simulink model "VT_Bridge"  (Simulink 7.5)
settings: Solver=ode45  StartTime=0.0  StopTime=10.0  RelTol=1e-3
libraries: powerlib x4
settings Model: Creator=lm  LastModifiedBy=lm

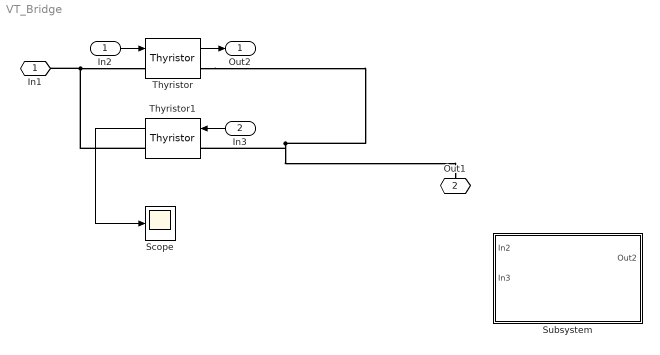
== system VT_Bridge ==
  In2 : Inport
  In3 : Inport  Port=2
  Scope : Scope
  Subsystem : Subsystem
  Thyristor : powerlib/Power Electronics/Thyristor  DialogController=POWERSYS.PowerSysDialog  SystemSampleTime=-1  Ron=0.001  Lon=0  Vf=0.8  IC=0  Rs=500  Cs=250e-9  Measurements=on
  Thyristor1 : powerlib/Power Electronics/Thyristor  DialogController=POWERSYS.PowerSysDialog  SystemSampleTime=-1  Ron=0.001  Lon=0  Vf=0.8  IC=0  Rs=500  Cs=250e-9  Measurements=on
  In1 : PMIOPort  Port=1  Side=Left
  Out1 : PMIOPort  Port=2  Side=Right
  Out2 : Outport
  wires:
  In3/1 -> Thyristor1/1
  Thyristor/1 -> Out2/1
  In2/1 -> Thyristor/1
  Thyristor1/1 -> Scope/1
  connections:
  Thyristor1/LConn1 -- Out1/RConn1 -- Thyristor/RConn1
  Thyristor1/RConn1 -- In1/RConn1 -- Thyristor/LConn1

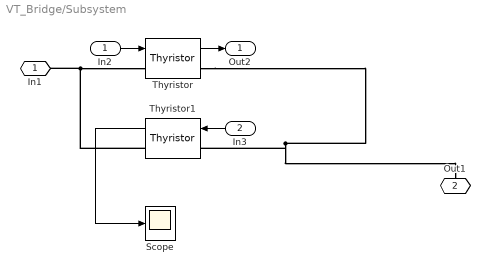
== system VT_Bridge/Subsystem ==
  In2 : Inport
  In3 : Inport  Port=2
  Scope : Scope
  Thyristor : powerlib/Power Electronics/Thyristor  DialogController=POWERSYS.PowerSysDialog  SystemSampleTime=-1  Ron=0.001  Lon=0  Vf=0.8  IC=0  Rs=500  Cs=250e-9  Measurements=on
  Thyristor1 : powerlib/Power Electronics/Thyristor  DialogController=POWERSYS.PowerSysDialog  SystemSampleTime=-1  Ron=0.001  Lon=0  Vf=0.8  IC=0  Rs=500  Cs=250e-9  Measurements=on
  In1 : PMIOPort  Port=1  Side=Left
  Out1 : PMIOPort  Port=2  Side=Right
  Out2 : Outport
  wires:
  In3/1 -> Thyristor1/1
  Thyristor/1 -> Out2/1
  In2/1 -> Thyristor/1
  Thyristor1/1 -> Scope/1
  connections:
  Thyristor1/LConn1 -- Thyristor/RConn1 -- Out1/RConn1
  Thyristor1/RConn1 -- Thyristor/LConn1 -- In1/RConn1
